simulink model "ISReferenceApplication"  (R2024b)
settings: Solver=ode4  StartTime=0.0  StopTime=60  FixedStep=1e-3  RelTol=5e-2
model workspace (MAT data in the model file):
  Downshift_Speeds = [9.5625 12.9375 16.3125 19.6875 23.0625 26.4375 29.8125 33.1875 36.5625 39.9375 43.3125 46.6875 ... (28 elements, 4x7)]
  EngRevLim = 7000
  Pedal_Positions = [0.1 0.4 0.5 0.9]
  Upshift_Speeds = [12.9375 16.3125 19.6875 33 26.4375 29.8125 33.1875 52.5 39.9375 43.3125 46.6875 77.25 ... (28 elements, 4x7)]
  VEH : object (value not decoded)
  rayDirections = [0 0 0 0 0 0 0 0 0 0 0 0 ... (363 elements, 121x3)]
  rayLengths = [20 20 20 20 20 20 20 20 20 20 20 20 ... (121 elements, 121x1)]
  rayOrigins = [0.5 0.4 0.3 0.2 0.1 0 -0.1 -0.2 -0.3 -0.4 -0.5 0.5 ... (363 elements, 121x3)]
  temp : object (value not decoded)
symbols that are objects in the model workspace (value not decoded): temp, VEH
undefined symbols (not defined in the file): DiscIntNeverNeededParam, Sim3dSensor
libraries: simulink x14, autolibutils x7, slpidlib x2, vehdynlibviscommon x2, sim3dgroundtruthsensorlib x2, autolibtranscontrolscommon x1, autolibshared x1, vehdynlibdriver x1, sharedtransform x1, vehdynlibsens x1, vehdynlibscenariocommon x1, sim3dlib x1
(part 4 of 4)

== matlab function ISReferenceApplication/Visualization/MATLAB Function ==
  data: pos input; agl input; vel input; wheel_agl input; T_ref input; track_w input; a input; b input; diameter input
function XYplot(pos,agl,vel,wheel_agl,T_ref,track_w,a,b,diameter)
persistent fig_xy ref_p
if isempty(fig_xy)
    fig_xy = figure();
    ref_p = plot(-T_ref(:,2),T_ref(:,1),'Color','red','LineWidth',1.5,'DisplayName','Ref. Path'); hold on;
end
body_yaw = agl(3);
body_x = pos(1);
body_y = pos(2);
wfl_x = body_x+a;
wfl_y = body_y-track_w/2;
wfr_x = body_x+a;
wfr_y = body_y+track_w/2;
wrl_x = body_x-b;
wrl_y = body_y-track_w/2;
wrr_x = body_x-b;
wrr_y = body_y+track_w/2;

R_whl = [cos(-wheel_agl(1)) -sin(-wheel_agl(1)) ;sin(-wheel_agl(1)) cos(-wheel_agl(1))];
R_bdy = [cos(-body_yaw) -sin(-body_yaw) ;sin(-body_yaw) cos(-body_yaw)];

wfl_rec_x = [wfl_y-0.1 wfl_y+0.1 wfl_y+0.1 wfl_y-0.1];
wfl_rec_y = [wfl_x-diameter/2 wfl_x-diameter/2 wfl_x+diameter/2 wfl_x+diameter/2];
wfr_rec_x = [wfr_y-0.1 wfr_y+0.1 wfr_y+0.1 wfr_y-0.1];
wfr_rec_y = [wfr_x-diameter/2 wfr_x-diameter/2 wfr_x+diameter/2 wfr_x+diameter/2];
wrl_rec_x = [wrl_y-0.1 wrl_y+0.1 wrl_y+0.1 wrl_y-0.1];
wrl_rec_y = [wrl_x-diameter/2 wrl_x-diameter/2 wrl_x+diameter/2 wrl_x+diameter/2];
wrr_rec_x = [wrr_y-0.1 wrr_y+0.1 wrr_y+0.1 wrr_y-0.1];
wrr_rec_y = [wrr_x-diameter/2 wrr_x-diameter/2 wrr_x+diameter/2 wrr_x+diameter/2];
bdy_rec_x = [body_y-1.731/2 body_y+1.731/2 body_y+1.731/2 body_y-1.731/2];
bdy_rec_y = [body_x-4.769/2 body_x-4.769/2 body_x+4.769/2 body_x+4.769/2];

wfl_rec = [wfl_rec_x;wfl_rec_y];
wfr_rec = [wfr_rec_x;wfr_rec_y];
wrl_rec = [wrl_rec_x;wrl_rec_y];
wrr_rec = [wrr_rec_x;wrr_rec_y];
bdy_rec = [bdy_rec_x;bdy_rec_y];

for i=1:4
    wfl_rec(:,i) = R_whl*(wfl_rec(:,i)-[wfl_y;wfl_x]) + [wfl_y;wfl_x];
    wfr_rec(:,i) = R_whl*(wfr_rec(:,i)-[wfr_y;wfr_x]) + [wfr_y;wfr_x];

    wfl_rec(:,i) = R_bdy*(wfl_rec(:,i)-[body_y;body_x]) + [body_y;body_x];
    wfr_rec(:,i) = R_bdy*(wfr_rec(:,i)-[body_y;body_x]) + [body_y;body_x];
    wrl_rec(:,i) = R_bdy*(wrl_rec(:,i)-[body_y;body_x]) + [body_y;body_x];
    wrr_rec(:,i) = R_bdy*(wrr_rec(:,i)-[body_y;body_x]) + [body_y;body_x];
    bdy_rec(:,i) = R_bdy*(bdy_rec(:,i)-[body_y;body_x]) + [body_y;body_x];
end

hold on;
bdy_sc = scatter(body_y,body_x,10,'black','filled','DisplayName','Trajectory');
txt = round(norm(vel(1:2))*3.6)+" km/h";
persistent wfl_p wfr_p wrl_p wrr_p bdy_p vel_p
if isempty(wfl_p)
    bdy_p = patch(bdy_rec(1,:),bdy_rec(2,:),'black','FaceAlpha',.5); hold on;
    wfl_p = patch(wfl_rec(1,:),wfl_rec(2,:),'black');
    wfr_p = patch(wfr_rec(1,:),wfr_rec(2,:),'black');
    wrl_p = patch(wrl_rec(1,:),wrl_rec(2,:),'black');
    wrr_p = patch(wrr_rec(1,:),wrr_rec(2,:),'black');
    vel_p = text(body_y-4,body_x+4,txt,'FontSize',11,'FontName','Arial');
else
    set(bdy_p,'XData',bdy_rec(1,:),'YData',bdy_rec(2,:));
    set(wfl_p,'XData',wfl_rec(1,:),'YData',wfl_rec(2,:));
    set(wfr_p,'XData',wfr_rec(1,:),'YData',wfr_rec(2,:));
    set(wrl_p,'XData',wrl_rec(1,:),'YData',wrl_rec(2,:));
    set(wrr_p,'XData',wrr_rec(1,:),'YData',wrr_rec(2,:));
    set(vel_p,'String',txt);
end

legend([ref_p,bdy_sc],{'Ref. Path','Trajectory'});

hold off;
axis('equal');
grid on;
ylim([body_x-(a+b)*2 body_x+(a+b)*2]);
xlim([body_y-(a+b)*2 body_y+(a+b)*2]);
xlabel('Y [m]'); ylabel('X [m]');

set(gca,'FontName','Arial','FontSize',11);

coder.extrinsic('F_Video');
F_Video();
end

== matlab function ISReferenceApplication/Driver Commands/MATLAB Function ==
  data: T_ref input; frntfromCG input; bdy_x input; bdy_y input; phi input; e output
function e = CrossTrackError(T_ref,frntfromCG,bdy_x,bdy_y,phi)
    % in case of center of grabity
    x = bdy_x;
    y = bdy_y;

    % in case of Front Axle
    frnt_axl = [cos(-phi) -sin(-phi); sin(-phi) cos(-phi)]*[frntfromCG;0];
    x = frnt_axl(1)+x;
    y = -frnt_axl(2)+y;

    d=.0;
    k=0;

    coder.extrinsic('F_CalcCrossTrackError');
    [d,k] = F_CalcCrossTrackError(T_ref,x,y);

    R = [cos(phi) -sin(phi); sin(phi) cos(phi)];
    r_ref = R*T_ref(k,1:2)';
    ego_ref = R*[x;-y];
    
    if ego_ref(2)<r_ref
        e=-d;
    else
        e=d;
    end
end

== matlab function ISReferenceApplication/Controllers/Brake Pressure Control/Bang Bang ABS/Kappa/MATLAB Function ==
  data: Omega input; xdot input; KappaEst output
function KappaEst = fcn(Omega, xdot)

Re = 0.29;
KappaEst = 0;
WhlSpd = Omega * Re;

if xdot*WhlSpd ~= 0
    KappaEst = (WhlSpd - xdot)/max([abs(xdot) abs(WhlSpd)]);
end

== matlab function ISReferenceApplication/Controllers/Brake Pressure Control/Five-State ABS and TCS/Wheel Accel and Slip Estimator/Kappa/MATLAB Function ==
  data: Omega input; xdot input; KappaEst output
function KappaEst = fcn(Omega, xdot)

Re = 0.29;
KappaEst = 0;
WhlSpd = Omega * Re;

if xdot*WhlSpd ~= 0
    KappaEst = (WhlSpd - xdot)/max([abs(xdot) abs(WhlSpd)]);
end

== stateflow chart ISReferenceApplication/Controllers/Brake Pressure Control/Five-State ABS and TCS/ABSCtrlForEach/For Each Subsystem/ABSForEachWheel ==
  state ABSOff
    entry:
    PbOutput = Pref;
    Flag = 0;
    during:
    PbOutput = Pref;
  state Normal
    entry:
    PbOutput = Pref;
    Flag = 0;
    during:
    PbOutput = Pref;
  state ABSOn
    state Phase1
      entry:
      PbOutput = v1;
      Flag = 1;
    state Phase5
      entry:
      PbOutput = v5;
      Flag = 5;
    state Phase2
      entry:
      PbOutput = 0;
      Flag = 2;
    state Phase4
      entry:
      PbOutput = 0;
      Flag = 4;
    state Phase3
      entry:
      PbOutput = v4;
      Flag = 3;
    (default) -> Phase1
    Phase5 -> Phase1 : [e2 < a2]
    Phase1 -> Phase2 : [e2 >= b]
    Phase4 -> Phase5 : [e2 <= a1]
    Phase2 -> Phase3 : [e2 >= A]
    Phase3 -> Phase4 : [e2 < A]
  (default) -> ABSOff
  ABSOn -> ABSOff : [abs(VehSpd) < 0.1 || Pref <= 0]
  Normal -> ABSOff [order 2] : [Pref <= 0]
  ABSOff -> Normal : [Pref > 0 && e2 < a2]
  Normal -> ABSOn [order 1] : [e1 < 0]
  data: e1 input; e2 input; PbOutput output; Flag output; b parameter; v1 parameter; v4 parameter; v5 parameter; A parameter; a2 parameter; a1 parameter; Pref input; VehSpd input
